simulink model "mortho_bpsk_1u_mp"  (Simulink 6.0)
settings: Solver=ode45  StartTime=0.0  StopTime=0.125 - (1/19200)  RelTol=1e-3
libraries: mspread x4, commchan2 x1, commsink2 x1, commseqgen2 x1, commrandsrc2 x1
CloseFcn:
  | clear spreadSigsOut
settings Model: Creator=akansal  LastModifiedBy=mmclerno  ProdHWDeviceType=Specified
settings DataIOCC: SaveTime=off  SignalLoggingName=spreadSigsOut
settings OptimizationCC: BooleanDataType=off  InlineParams=on  MultiInstanced=off
settings FormatCC: IgnoreBidirectionalLines=off
settings HardwareCC: ProdHWDeviceType=Specified
settings CodeAppCC: SimulinkBlockComments=off
settings GRTTargetCC: TargetFcnLib=iso_c_tmw.mat

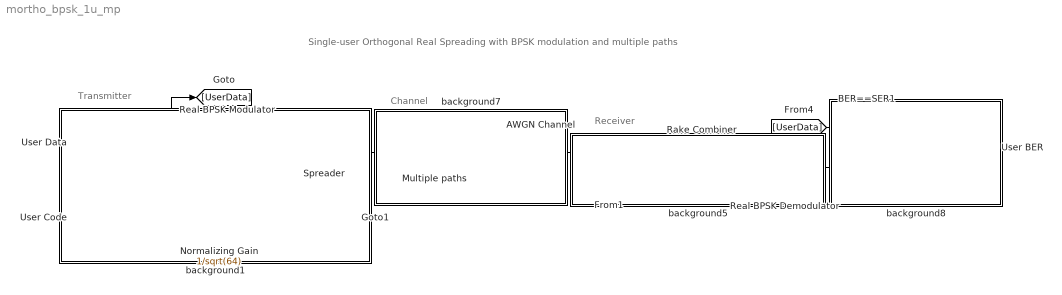
== system mortho_bpsk_1u_mp ==
  note: Single-user Orthogonal Real Spreading with BPSK modulation and multiple paths
  note: Transmitter
  note: Channel
  note: Receiver
  AWGN Channel : commchan2/AWGN Channel  seed=1237  noiseMode="Signal to noise ratio  (SNR)"  EbNodB=10  EsNodB=25  SNRdB=5  bitsPerSym=1  Ps=1  Tsym=ts  variance=1
  BER==SER1 : commsink2/Error Rate Calculation  N=0  st_delay=0  cp_mode=Entire frame  subframe=[]  PMode=Port  WsName=ErrorVec  RsMode2=off  stop=off  numErr=100  maxBits=1e6
  Multiple paths : mspread/Multiple paths  p=3  pd=[0 3 5]  ts=1/19200
  Normalizing Gain : Gain  Gain=1/sqrt(64)  SaturateOnIntegerOverflow=on
  Rake Combiner : mspread/Rake Combiner  pd=[0 3 5]  pgain=64
  Real BPSK Demodulator : mspread/Real BPSK Demodulator
  Real BPSK Modulator : mspread/Real BPSK Modulator
  Spreader : Product  SaturateOnIntegerOverflow=on  InputSameDT=on
  User BER : Display
  User Code : commseqgen2/Hadamard Code Generator  length=64  index=30  ts=1/(19200*64)  frameBased=on  sampPerFrame=64
  User Data : commrandsrc2/Random Integer Generator  mul=2  seed=631  Ts=1/19200  frameBased=on  sampPerFrame=1  orient=off
  background1 : Subsystem
      mask Display: disp('')
  background5 : Subsystem
      mask Display: disp('')
  background7 : Subsystem  Orientation=up
      mask Display: disp('')
  background8 : Subsystem
      mask Display: disp('')
  wires:
  User Data/1 -> [UserData], Real BPSK Modulator/1
  Real BPSK Modulator/1 -> Spreader/1
  Spreader/1 -> Multiple paths/1
  User Code/1 -> Normalizing Gain/1
  Normalizing Gain/1 -> Spreader/2, [UserCode]
  AWGN Channel/1 -> Rake Combiner/1
  Multiple paths/1 -> AWGN Channel/1
  [UserCode] -> Rake Combiner/2
  Real BPSK Demodulator/1 -> BER==SER1/2
  [UserData] -> BER==SER1/1
  BER==SER1/1 -> User BER/1
  Rake Combiner/1 -> Real BPSK Demodulator/1

== system mortho_bpsk_1u_mp/background1 ==

== system mortho_bpsk_1u_mp/background5 ==

== system mortho_bpsk_1u_mp/background7 ==

== system mortho_bpsk_1u_mp/background8 ==
